simulink subsystem "NoEngine"  (R2022b)
settings: Solver=VariableStepAuto  StartTime=0.0  StopTime=10.0  RelTol=1e-3
settings Model: Creator=The MathWorks, Inc.  LastModifiedBy=The MathWorks, Inc.

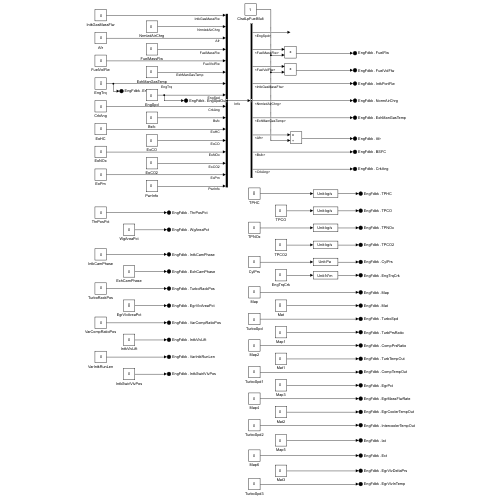
[thumbnail: Simulink's stored preview of the top-level diagram]
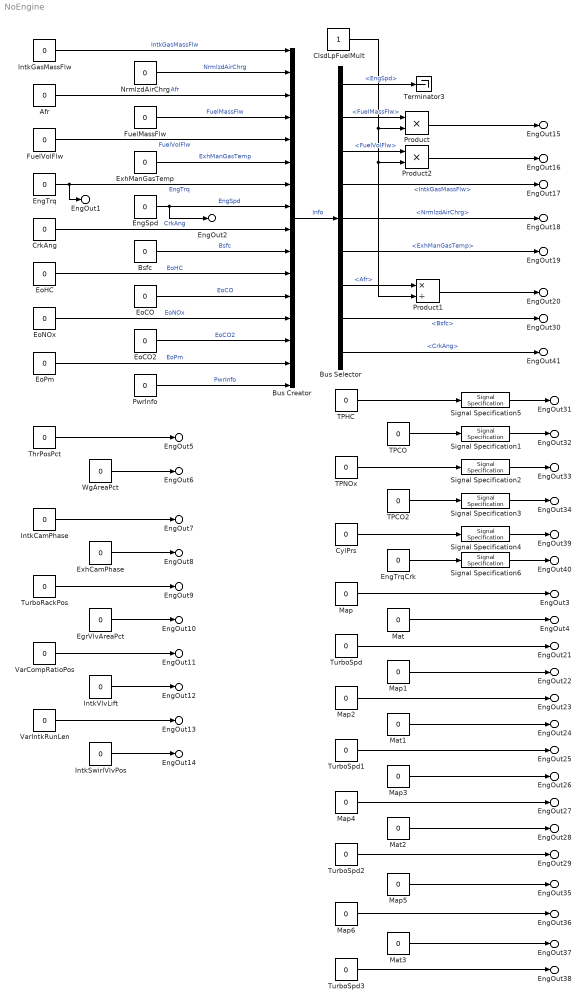
== system NoEngine ==
  Afr : Constant  Value=0  SampleTime=-1
  Bsfc : Constant  Value=0  SampleTime=-1
  Bus Creator : BusCreator  Inputs=16
  Bus Selector : BusSelector  OutputSignals=EngSpd,FuelMassFlw,FuelVolFlw,IntkGasMassFlw,NrmlzdAirChrg,ExhManGasTemp,Afr,Bsfc,CrkAng
  ClsdLpFuelMult : Constant  SampleTime=-1
  CrkAng : Constant  Value=0  SampleTime=-1
  CylPrs : Constant  Value=0  SampleTime=-1
  EgrVlvAreaPct : Constant  Value=0  SampleTime=-1
  EngSpd : Constant  Value=0  SampleTime=-1
  EngTrq : Constant  Value=0  SampleTime=-1
  EngTrqCrk : Constant  Value=0  SampleTime=-1
  EoCO : Constant  Value=0  SampleTime=-1
  EoCO2 : Constant  Value=0  SampleTime=-1
  EoHC : Constant  Value=0  SampleTime=-1
  EoNOx : Constant  Value=0  SampleTime=-1
  EoPm : Constant  Value=0  SampleTime=-1
  ExhCamPhase : Constant  Value=0  SampleTime=-1
  ExhManGasTemp : Constant  Value=0  SampleTime=-1
  FuelMassFlw : Constant  Value=0  SampleTime=-1
  FuelVolFlw : Constant  Value=0  SampleTime=-1
  IntkCamPhase : Constant  Value=0  SampleTime=-1
  IntkGasMassFlw : Constant  Value=0  SampleTime=-1
  IntkSwirlVlvPos : Constant  Value=0  SampleTime=-1
  IntkVlvLift : Constant  Value=0  SampleTime=-1
  Map{,1..6} (7 alike) : Constant  Value=0  SampleTime=-1
  Mat{,1..3} (4 alike) : Constant  Value=0  SampleTime=-1
  NrmlzdAirChrg : Constant  Value=0  SampleTime=-1
  Product : Product
  Product1 : Product  Inputs=*/
  Product2 : Product
  PwrInfo : Constant  Value=0  SampleTime=-1
  Signal Specification{1..3,5} (4 alike) : SignalSpecification  Unit=kg/s
  Signal Specification4 : SignalSpecification  Unit=Pa
  Signal Specification6 : SignalSpecification  Unit=N*m
  TPCO : Constant  Value=0  SampleTime=-1
  TPCO2 : Constant  Value=0  SampleTime=-1
  TPHC : Constant  Value=0  SampleTime=-1
  TPNOx : Constant  Value=0  SampleTime=-1
  Terminator3 : Terminator
  ThrPosPct : Constant  Value=0  SampleTime=-1
  TurboRackPos : Constant  Value=0  SampleTime=-1
  TurboSpd{,1..3} (4 alike) : Constant  Value=0  SampleTime=-1
  VarCompRatioPos : Constant  Value=0  SampleTime=-1
  VarIntkRunLen : Constant  Value=0  SampleTime=-1
  WgAreaPct : Constant  Value=0  SampleTime=-1
  EngOut1 : Outport  PortName=EngFdbk  Element=EngTrq
  EngOut2 : Outport  PortName=EngFdbk  Element=EngSpdOut
  EngOut3 : Outport  PortName=EngFdbk  Element=Map
  EngOut4 : Outport  PortName=EngFdbk  Element=Mat
  EngOut5 : Outport  PortName=EngFdbk  Element=ThrPosPct
  EngOut6 : Outport  PortName=EngFdbk  Element=WgAreaPct
  EngOut7 : Outport  PortName=EngFdbk  Element=IntkCamPhase
  EngOut8 : Outport  PortName=EngFdbk  Element=ExhCamPhase
  EngOut9 : Outport  PortName=EngFdbk  Element=TurboRackPos
  EngOut10 : Outport  PortName=EngFdbk  Element=EgrVlvAreaPct
  EngOut11 : Outport  PortName=EngFdbk  Element=VarCompRatioPos
  EngOut12 : Outport  PortName=EngFdbk  Element=IntkVlvLift
  EngOut13 : Outport  PortName=EngFdbk  Element=VarIntkRunLen
  EngOut14 : Outport  PortName=EngFdbk  Element=IntkSwirlVlvPos
  EngOut15 : Outport  PortName=EngFdbk  Element=FuelFlw
  EngOut16 : Outport  PortName=EngFdbk  Element=FuelVolFlw
  EngOut17 : Outport  PortName=EngFdbk  Element=IntkPortFlw
  EngOut18 : Outport  PortName=EngFdbk  Element=NormAirChrg
  EngOut19 : Outport  PortName=EngFdbk  Element=ExhManGasTemp
  EngOut20 : Outport  PortName=EngFdbk  Element=Afr
  EngOut21 : Outport  PortName=EngFdbk  Element=TurboSpd
  EngOut22 : Outport  PortName=EngFdbk  Element=TurbPrsRatio
  EngOut23 : Outport  PortName=EngFdbk  Element=CompPrsRatio
  EngOut24 : Outport  PortName=EngFdbk  Element=TurbTempOut
  EngOut25 : Outport  PortName=EngFdbk  Element=CompTempOut
  EngOut26 : Outport  PortName=EngFdbk  Element=EgrPct
  EngOut27 : Outport  PortName=EngFdbk  Element=EgrMassFlwRate
  EngOut28 : Outport  PortName=EngFdbk  Element=EgrCoolerTempOut
  EngOut29 : Outport  PortName=EngFdbk  Element=IntercoolerTempOut
  EngOut30 : Outport  PortName=EngFdbk  Element=BSFC
  EngOut31 : Outport  PortName=EngFdbk  Element=TPHC
  EngOut32 : Outport  PortName=EngFdbk  Element=TPCO
  EngOut33 : Outport  PortName=EngFdbk  Element=TPNOx
  EngOut34 : Outport  PortName=EngFdbk  Element=TPCO2
  EngOut35 : Outport  PortName=EngFdbk  Element=Iat
  EngOut36 : Outport  PortName=EngFdbk  Element=Ect
  EngOut37 : Outport  PortName=EngFdbk  Element=EgrVlvDeltaPrs
  EngOut38 : Outport  PortName=EngFdbk  Element=EgrVlvInTemp
  EngOut39 : Outport  PortName=EngFdbk  Element=CylPrs
  EngOut40 : Outport  PortName=EngFdbk  Element=EngTrqCrk
  EngOut41 : Outport  PortName=EngFdbk  Element=CrkAng
  wires:
  ClsdLpFuelMult/1 -> Product/2, Product1/2, Product2/2
  CrkAng/1 -> Bus Creator/9  "CrkAng"
  Map2/1 -> EngOut23/1
  Map3/1 -> EngOut26/1
  EoCO2/1 -> Bus Creator/14  "EoCO2"
  TurboSpd1/1 -> EngOut25/1
  Map6/1 -> EngOut36/1
  FuelMassFlw/1 -> Bus Creator/4  "FuelMassFlw"
  Bus Selector/4 -> EngOut17/1  "<IntkGasMassFlw>"
  Signal Specification5/1 -> EngOut31/1
  Mat3/1 -> EngOut37/1
  Signal Specification4/1 -> EngOut39/1
  Product2/1 -> EngOut16/1
  IntkGasMassFlw/1 -> Bus Creator/1  "IntkGasMassFlw"
  Map5/1 -> EngOut35/1
  TPNOx/1 -> Signal Specification2/1
  TPHC/1 -> Signal Specification5/1
  CylPrs/1 -> Signal Specification4/1
  Signal Specification3/1 -> EngOut34/1
  Mat2/1 -> EngOut28/1
  Bus Selector/8 -> EngOut30/1  "<Bsfc>"
  VarCompRatioPos/1 -> EngOut11/1
  ThrPosPct/1 -> EngOut5/1
  Bus Selector/2 -> Product/1  "<FuelMassFlw>"
  TurboRackPos/1 -> EngOut9/1
  Map1/1 -> EngOut22/1
  VarIntkRunLen/1 -> EngOut13/1
  WgAreaPct/1 -> EngOut6/1
  Bus Selector/3 -> Product2/1  "<FuelVolFlw>"
  EngTrqCrk/1 -> Signal Specification6/1
  Signal Specification1/1 -> EngOut32/1
  TurboSpd3/1 -> EngOut38/1
  Mat/1 -> EngOut4/1
  IntkSwirlVlvPos/1 -> EngOut14/1
  IntkVlvLift/1 -> EngOut12/1
  Bus Selector/6 -> EngOut19/1  "<ExhManGasTemp>"
  ExhCamPhase/1 -> EngOut8/1
  Product1/1 -> EngOut20/1
  Bus Selector/7 -> Product1/1  "<Afr>"
  TPCO2/1 -> Signal Specification3/1
  Afr/1 -> Bus Creator/3  "Afr"
  EoHC/1 -> Bus Creator/11  "EoHC"
  Map/1 -> EngOut3/1
  Signal Specification6/1 -> EngOut40/1
  EoPm/1 -> Bus Creator/15  "EoPm"
  Bus Selector/9 -> EngOut41/1  "<CrkAng>"
  TurboSpd2/1 -> EngOut29/1
  IntkCamPhase/1 -> EngOut7/1
  EngTrq/1 -> Bus Creator/7, EngOut1/1  "EngTrq"
  Bus Creator/1 -> Bus Selector/1  "Info"
  Signal Specification2/1 -> EngOut33/1
  Bus Selector/5 -> EngOut18/1  "<NrmlzdAirChrg>"
  Map4/1 -> EngOut27/1
  PwrInfo/1 -> Bus Creator/16  "PwrInfo"
  Mat1/1 -> EngOut24/1
  TPCO/1 -> Signal Specification1/1
  Product/1 -> EngOut15/1
  FuelVolFlw/1 -> Bus Creator/5  "FuelVolFlw"
  NrmlzdAirChrg/1 -> Bus Creator/2  "NrmlzdAirChrg"
  ExhManGasTemp/1 -> Bus Creator/6  "ExhManGasTemp"
  Bsfc/1 -> Bus Creator/10  "Bsfc"
  TurboSpd/1 -> EngOut21/1
  EgrVlvAreaPct/1 -> EngOut10/1
  Bus Selector/1 -> Terminator3/1  "<EngSpd>"
  EoCO/1 -> Bus Creator/12  "EoCO"
  EngSpd/1 -> EngOut2/1, Bus Creator/8  "EngSpd"
  EoNOx/1 -> Bus Creator/13  "EoNOx"
